simulink model "W1_P9"  (R2020b)
settings: Solver=VariableStepAuto  StartTime=0.0  StopTime=10.0  RelTol=1e-3
libraries: simulink x1, pid_lib x1
settings Model: Creator=ADMIN  LastModifiedBy=ADMIN

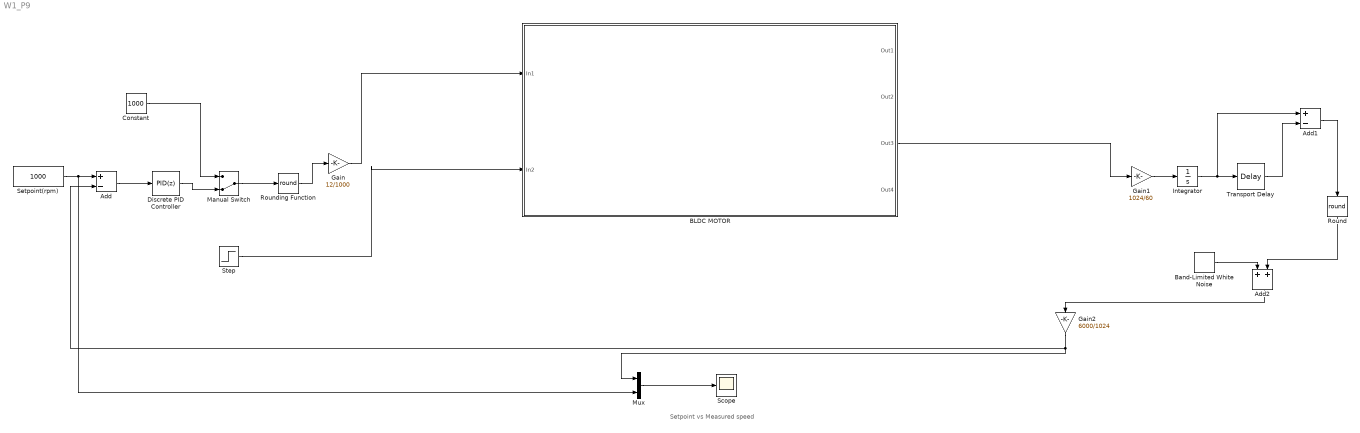
== system W1_P9 ==
  note: Setpoint vs Measured speed
  Add : Sum  Inputs=+-
  Add1 : Sum  Inputs=+-
  Add2 : Sum
  BLDC MOTOR : Subsystem
  Band-Limited White Noise : simulink/Sources/Band-Limited White Noise  Cov=[0.1]  Ts=0.1  seed=[23341]
  Constant : Constant  Value=1000
  Discrete PID Controller : pid_lib/PID Controller  Controller=PID  Form=Parallel  TimeDomain=Discrete-time  UseExternalTs=off  SampleTime=-1  IntegratorMethod=Forward Euler  FilterMethod=Forward Euler  ControllerParametersSource=internal  P=1  I=1  D=0  UseFilter=on  N=100  TunerSelectOption=Transfer Function Based (PID Tuner App)  InitialConditionSource=internal  InitialConditionForIntegrator=0  InitialConditionForFilter=0  DifferentiatorICPrevScaledInput=0  ExternalReset=none  TrackingMode=off  Kt=1  LimitOutput=off  SatLimitsSource=internal  UpperSaturationLimit=inf  LowerSaturationLimit=-inf  LinearizeAsGain=off  AntiWindupMode=none  Kb=1  POutMin=[]  POutMax=[]  IOutMin=[]  IOutMax=[]  DOutMin=[]  DOutMax=[]  NOutMin=[]  NOutMax=[]  SumOutMin=[]  SumOutMax=[]  SaturationOutMin=[]  SaturationOutMax=[]  PParamMin=[]  PParamMax=[]  IParamMin=[]  IParamMax=[]  DParamMin=[]  DParamMax=[]  NParamMin=[]  NParamMax=[]  KbParamMin=[]  KbParamMax=[]  KtParamMin=[]  KtParamMax=[]  KbOutMin=[]  KbOutMax=[]  KtOutMin=[]  KtOutMax=[]  IntegratorOutMin=[]  IntegratorOutMax=[]  FilterOutMin=[]  FilterOutMax=[]  SumI1OutMin=[]  SumI1OutMax=[]  SumI2OutMin=[]  SumI2OutMax=[]  SumI3OutMin=[]  SumI3OutMax=[]  SumI4OutMin=[]  SumI4OutMax=[]  SumDOutMin=[]  SumDOutMax=[]  DifferentiatorOutMin=[]  DifferentiatorOutMax=[]  FilterDiffOutCoefMin=[]  FilterDiffOutCoefMax=[]  ReciprocalOutMin=[]  ReciprocalOutMax=[]  SumDenOutMin=[]  SumDenOutMax=[]  SumNumOutMin=[]  SumNumOutMax=[]  DivideOutMin=[]  DivideOutMax=[]  UdiffTsProdOutMin=[]  UdiffTsProdOutMax=[]  NTsProdOutMin=[]  NTsProdOutMax=[]  UintegralTsProdOutMin=[]  UintegralTsProdOutMax=[]  UngainTsProdOutMin=[]  UngainTsProdOutMax=[]  IntegratorContinuousStateAttributes=''  IntegratorStateMustResolveToSignalObject=off  IntegratorRTWStateStorageClass=Auto  FilterContinuousStateAttributes=''  FilterStateMustResolveToSignalObject=off  FilterRTWStateStorageClass=Auto  ParallelPVariant=InternalParameters  IdealPVariant=Disabled  IVariant=InternalParameters  DVariant=InternalParameters  IntegratorVariant=Discrete  SatVariant=Disabled  AWVariant=Passthrough  PCopyVariant=Disabled  TRVariant=Disabled  FdbkBlocksVariant=Forward  IdealPFdbkVariant=Disabled  SatFdbkVariant=Disabled  DerivativeFilterVariant=ForwardEulerFilter  NVariant=InternalParameters  NCopyVariant=Disabled  FilterICVariant=InternalICsFilter  IntegratorICVariant=InternalICs  ExternalResetVariant=Disabled  TRSumVariant=Passthrough  SumFdbkVariant=Disabled  SumVariant=Sum_PID  TsampFilterVariant=InternalTs  TsampNgainVariant=Passthrough  TsampIntegralVariant=Passthrough  ExternalSaturationOutDataTypeStr=Inherit: Same as second input
  Gain : Gain  Gain=12/1000
  Gain1 : Gain  Gain=1024/60
  Gain2 : Gain  Gain=6000/1024
  Integrator : Integrator
  Manual Switch : ManualSwitch  CurrentSetting=0
  Mux : Mux  Inputs=2
  Round : Rounding  Operator=round
  Rounding Function : Rounding  Operator=round
  Scope : Scope
  Setpoint(rpm) : Constant  Value=1000
  Step : Step  SampleTime=0
  Transport Delay : TransportDelay
  wires:
  Rounding Function/1 -> Gain/1
  Transport Delay/1 -> Add1/2
  Integrator/1 -> Add1/1, Transport Delay/1
  Add1/1 -> Round/1
  Gain1/1 -> Integrator/1
  Constant/1 -> Manual Switch/1
  Mux/1 -> Scope/1
  Manual Switch/1 -> Rounding Function/1
  Add/1 -> Discrete PID Controller/1
  Setpoint(rpm)/1 -> Mux/2, Add/1
  Add2/1 -> Gain2/1
  Gain2/1 -> Mux/1, Add/2
  Round/1 -> Add2/2
  Band-Limited White Noise/1 -> Add2/1
  Discrete PID Controller/1 -> Manual Switch/2
  Gain/1 -> BLDC MOTOR/1(In1)
  Step/1 -> BLDC MOTOR/2(In2)
  BLDC MOTOR/3(Out3) -> Gain1/1

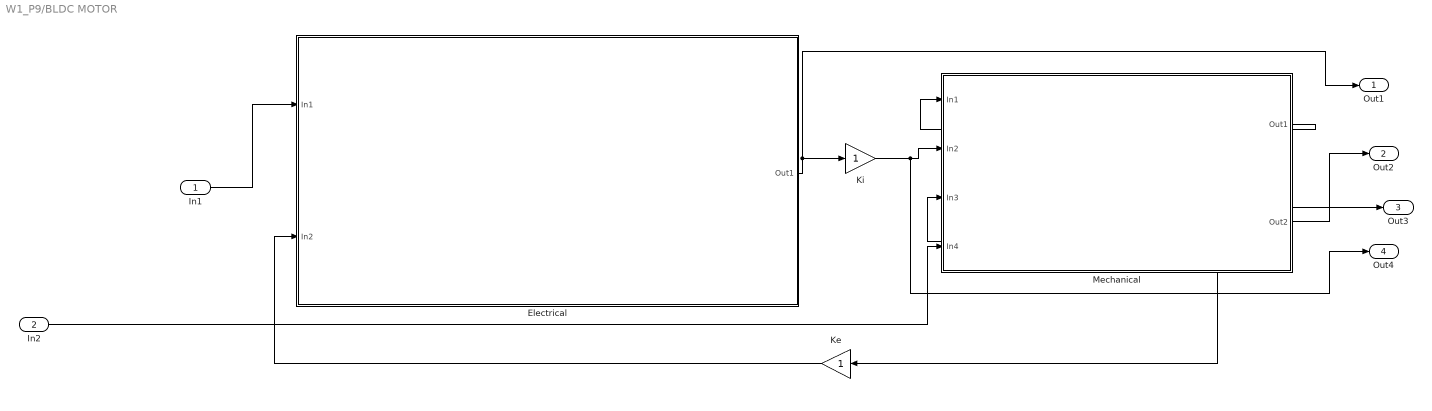
== system W1_P9/BLDC MOTOR ==
  In1 : Inport
  In2 : Inport  Port=2
  Electrical : Subsystem
  Ke : Gain
  Ki : Gain
  Mechanical : Subsystem
  Out1 : Outport
  Out2 : Outport  Port=2
  Out3 : Outport  Port=3
  Out4 : Outport  Port=4
  wires:
  Ki/1 -> Mechanical/2(In2), Out4/1
  Electrical/1(Out1) -> Out1/1, Ki/1
  In1/1 -> Electrical/1(In1)
  Ke/1 -> Electrical/2(In2)
  Mechanical/1(Out1) -> Mechanical/1(In1), Mechanical/3(In3), Ke/1, Out3/1
  In2/1 -> Mechanical/4(In4)
  Mechanical/2(Out2) -> Out2/1

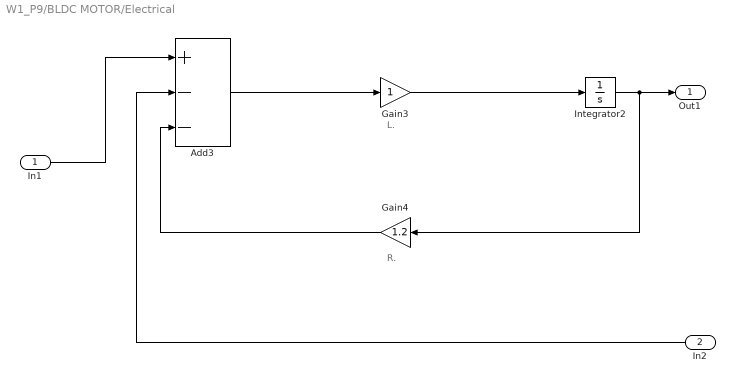
== system W1_P9/BLDC MOTOR/Electrical ==
  note: L.
  note: R.
  In1 : Inport
  In2 : Inport  Port=2
  Add3 : Sum  Inputs=+--
  Gain3 : Gain
  Gain4 : Gain  Gain=1.2
  Integrator2 : Integrator
  Out1 : Outport
  wires:
  Integrator2/1 -> Out1/1, Gain4/1
  Gain3/1 -> Integrator2/1
  In1/1 -> Add3/1
  Gain4/1 -> Add3/3
  In2/1 -> Add3/2
  Add3/1 -> Gain3/1

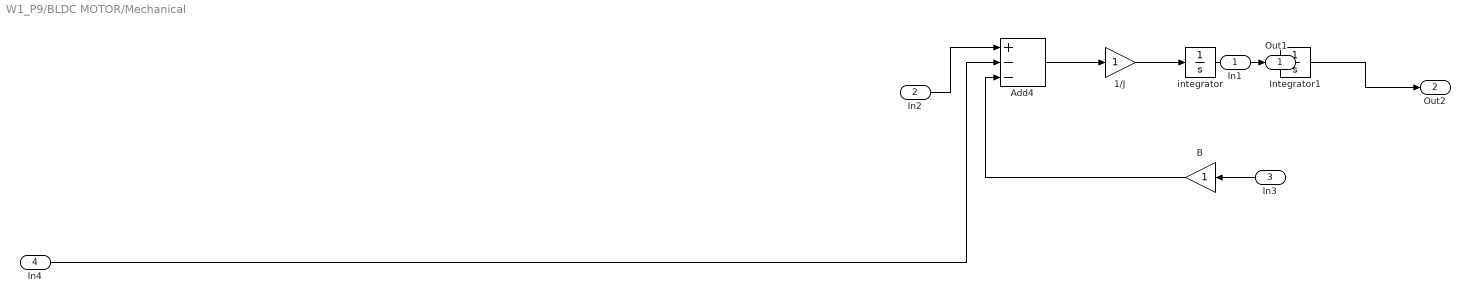
== system W1_P9/BLDC MOTOR/Mechanical ==
  In1 : Inport
  In2 : Inport  Port=2
  In3 : Inport  Port=3
  In4 : Inport  Port=4
  1/J : Gain
  Add4 : Sum  Inputs=+--
  B : Gain
  Integrator1 : Integrator
  integrator : Integrator
  Out1 : Outport
  Out2 : Outport  Port=2
  wires:
  integrator/1 -> Out1/1
  Add4/1 -> 1/J/1
  1/J/1 -> integrator/1
  In2/1 -> Add4/1
  B/1 -> Add4/3
  In1/1 -> Integrator1/1
  In3/1 -> B/1
  In4/1 -> Add4/2
  Integrator1/1 -> Out2/1
